simulink subsystem "BEVController_refsub_Basic"  (R2023a)
settings: Solver=VariableStepAuto  StartTime=0.0  StopTime=10.0  RelTol=1e-3
undefined symbols (not defined in the file): bevControl
libraries: rllib x1
settings Model: Creator=isaacito  LastModifiedBy=tu101
settings OptimizationCC: ReuseModelBlockBuffer=off

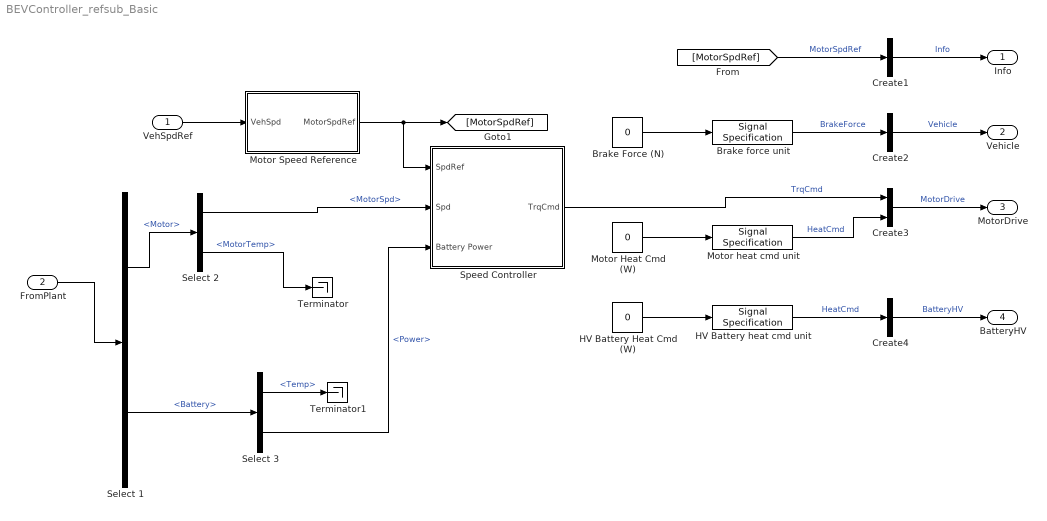
== system BEVController_refsub_Basic ==
  VehSpdRef : Inport
  FromPlant : Inport  Port=2
  Brake Force (N) : Constant  Value=0
  Brake force unit : SignalSpecification  Unit=N
  Create1 : BusCreator  Inputs=1
  Create2 : BusCreator  Inputs=1
  Create3 : BusCreator  Inputs=2
  Create4 : BusCreator  Inputs=1
  HV Battery Heat Cmd (W) : Constant  Value=0
  HV Battery heat cmd unit : SignalSpecification  Unit=W
  Motor Heat Cmd (W) : Constant  Value=0
  Motor Speed Reference : Subsystem
  Motor heat cmd unit : SignalSpecification  Unit=W
  Select 1 : BusSelector  OutputSignals=Motor,Battery
  Select 2 : BusSelector  OutputSignals=MotorSpd,MotorTemp
  Select 3 : BusSelector  OutputSignals=Temp,Power
  Speed Controller : Subsystem
  Terminator : Terminator
  Terminator1 : Terminator
  Info : Outport
  Vehicle : Outport  Port=2
  MotorDrive : Outport  Port=3
  BatteryHV : Outport  Port=4
  wires:
  Motor Speed Reference/1(MotorSpdRef) -> [MotorSpdRef], Speed Controller/1(SpdRef)
  Select 2/1 -> Speed Controller/2(Spd)  "<MotorSpd>"
  VehSpdRef/1 -> Motor Speed Reference/1(VehSpd)
  Brake Force (N)/1 -> Brake force unit/1
  FromPlant/1 -> Select 1/1
  Select 1/1 -> Select 2/1  "<Motor>"
  [MotorSpdRef] -> Create1/1  "MotorSpdRef"
  Create1/1 -> Info/1  "Info"
  Create2/1 -> Vehicle/1  "Vehicle"
  Create3/1 -> MotorDrive/1  "MotorDrive"
  Create4/1 -> BatteryHV/1  "BatteryHV"
  Select 1/2 -> Select 3/1  "<Battery>"
  Motor Heat Cmd (W)/1 -> Motor heat cmd unit/1
  HV Battery Heat Cmd (W)/1 -> HV Battery heat cmd unit/1
  Select 2/2 -> Terminator/1  "<MotorTemp>"
  Select 3/1 -> Terminator1/1  "<Temp>"
  Motor heat cmd unit/1 -> Create3/2  "HeatCmd"
  HV Battery heat cmd unit/1 -> Create4/1  "HeatCmd"
  Brake force unit/1 -> Create2/1  "BrakeForce"
  Speed Controller/1(TrqCmd) -> Create3/1  "TrqCmd"
  Select 3/2 -> Speed Controller/3(Battery Power)  "<Power>"

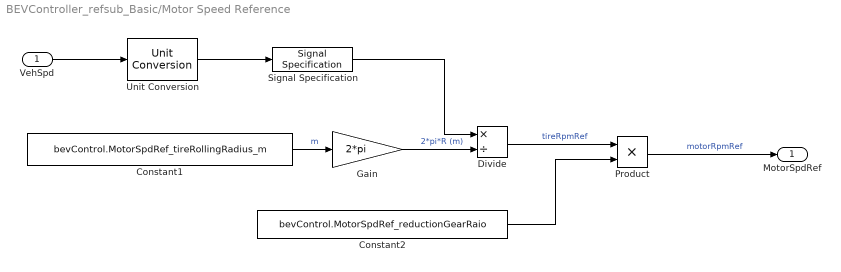
== system BEVController_refsub_Basic/Motor Speed Reference ==
  VehSpd : Inport  Unit=km/hr
  Constant1 : Constant  Value=bevControl.MotorSpdRef_tireRollingRadius_m
  Constant2 : Constant  Value=bevControl.MotorSpdRef_reductionGearRaio
  Divide : Product  Inputs=*/
  Gain : Gain  Gain=2*pi
  Product : Product
  Signal Specification : SignalSpecification  Unit=m/min
  Unit Conversion : UnitConversion
  MotorSpdRef : Outport  Unit=rpm  VectorParamsAs1DForOutWhenUnconnected=off
  wires:
  Constant1/1 -> Gain/1  "m"
  Product/1 -> MotorSpdRef/1  "motorRpmRef"
  Constant2/1 -> Product/2
  Divide/1 -> Product/1  "tireRpmRef"
  Gain/1 -> Divide/2  "2*pi*R (m)"
  Signal Specification/1 -> Divide/1
  Unit Conversion/1 -> Signal Specification/1
  VehSpd/1 -> Unit Conversion/1

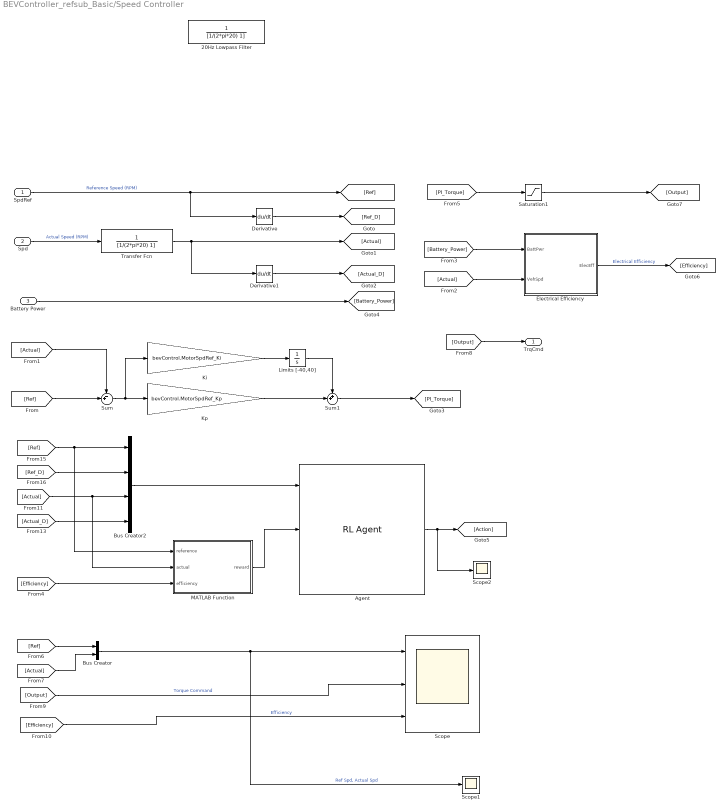
== system BEVController_refsub_Basic/Speed Controller ==
  SpdRef : Inport  Unit=rpm
      settings: AttributesFormatString=%<Unit>
  Spd : Inport  Port=2  Unit=rpm
      settings: AttributesFormatString=%<Unit>
  Battery Power : Inport  Port=3  Unit=kW
  20Hz Lowpass Filter : TransferFcn  Denominator=[1/(2*pi*20) 1]
  Agent : rllib/RL Agent  Agent=RL_Agent_0608  ExternalActionAsInput=off  ProvideLastAction=off  ProvideCumRwd=off  TreatAsDirectFeedthrough=on  UseStrictObservationDataTypes=off
  Bus Creator : BusCreator  Inputs=2
  Bus Creator2 : BusCreator  Inputs=4
  Derivative : Derivative
  Derivative1 : Derivative
  Electrical Efficiency : Subsystem
  Ki : Gain  Gain=bevControl.MotorSpdRef_Ki
  Kp : Gain  Gain=bevControl.MotorSpdRef_Kp
  Limits [-40,40] : Integrator  LimitOutput=on  UpperSaturationLimit=40  LowerSaturationLimit=-40
  MATLAB Function : MATLAB Function  TreatAsAtomicUnit=on
  Saturation1 : Saturate  UpperLimit=bevControl.MotorDriveUnit_trqMax_Nm  LowerLimit=-bevControl.MotorDriveUnit_trqMax_Nm
      settings: AttributesFormatString=|
      | %<UpperLimit>
      | %<LowerLimit>
  Scope : Scope  NumInputPorts=3
  Scope1 : Scope
  Scope2 : Scope
  Sum : Sum  Inputs=-+|
  Sum1 : Sum  Inputs=++|
  Transfer Fcn : TransferFcn  Denominator=[1/(2*pi*20) 1]
  TrqCmd : Outport  Unit=N*m  VectorParamsAs1DForOutWhenUnconnected=off
      settings: AttributesFormatString=%<Unit>
  wires:
  [Output] -> Scope/2  "Torque Command"
  [Output] -> TrqCmd/1
  [Actual] -> Bus Creator/2
  Bus Creator/1 -> Scope/1, Scope1/1  "Ref Spd, Actual Spd"
  [Ref] -> Bus Creator/1
  Transfer Fcn/1 -> [Actual], Derivative1/1
  Spd/1 -> Transfer Fcn/1  "Actual Speed (RPM)"
  [Efficiency] -> Scope/3  "Efficiency"
  [Efficiency] -> MATLAB Function/3(efficiency)
  Electrical Efficiency/1(ElecEff) -> [Efficiency]  "Electrical Efficiency"
  Battery Power/1 -> [Battery_Power]
  [Actual] -> Electrical Efficiency/2(VehSpd)
  [Actual] -> Sum/1
  [Ref] -> Sum/2
  [Battery_Power] -> Electrical Efficiency/1(BattPwr)
  MATLAB Function/1(reward) -> Agent/2
  Bus Creator2/1 -> Agent/1
  [Actual_D] -> Bus Creator2/4
  [Actual] -> Bus Creator2/3, MATLAB Function/2(actual)
  [Ref] -> Bus Creator2/1, MATLAB Function/1(reference)
  [Ref_D] -> Bus Creator2/2
  Agent/1 -> [Action], Scope2/1
  Saturation1/1 -> [Output]
  [PI_Torque] -> Saturation1/1
  Derivative1/1 -> [Actual_D]
  Derivative/1 -> [Ref_D]
  SpdRef/1 -> [Ref], Derivative/1  "Reference Speed (RPM)"
  Sum1/1 -> [PI_Torque]
  Sum/1 -> Ki/1, Kp/1
  Ki/1 -> Limits [-40,40]/1
  Kp/1 -> Sum1/2
  Limits [-40,40]/1 -> Sum1/1

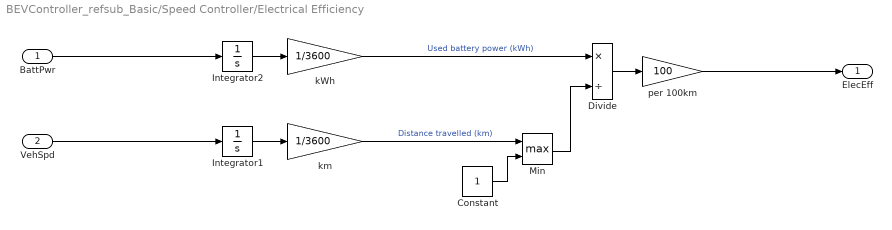
== system BEVController_refsub_Basic/Speed Controller/Electrical Efficiency ==
  BattPwr : Inport  Unit=kW
  VehSpd : Inport  Port=2  Unit=km/hr
  Constant : Constant
  Divide : Product  Inputs=*/
  Integrator1 : Integrator
  Integrator2 : Integrator
  Min : MinMax  Function=max  Inputs=2
  kWh : Gain  Gain=1/3600
  km : Gain  Gain=1/3600
  per 100km : Gain  Gain=100
  ElecEff : Outport  Unit=kW*hr/(100*km)
  wires:
  VehSpd/1 -> Integrator1/1
  BattPwr/1 -> Integrator2/1
  per 100km/1 -> ElecEff/1
  kWh/1 -> Divide/1  "Used battery power (kWh)"
  Min/1 -> Divide/2
  Integrator1/1 -> km/1
  Divide/1 -> per 100km/1
  Integrator2/1 -> kWh/1
  Constant/1 -> Min/2
  km/1 -> Min/1  "Distance travelled (km)"

== matlab function BEVController_refsub_Basic/Speed Controller/MATLAB Function ==
  data: reference input; reward output; actual input; efficiency input
function reward = calReward(reference, actual, efficiency)

reward = -100 * abs(reference - actual);
